simulink model "particle_fluid_surface_interaction_model"  (R2024b)
settings: Solver=ode4  StartTime=0.0  StopTime=params.tEnd  FixedStep=params.dt  RelTol=1e-3
undefined symbols (not defined in the file): params
libraries: slpidlib x1
settings Model: Creator=nihalseth34  LastModifiedBy=nihalseth34
settings DebuggingCC: AlgebraicLoopMsg=none  IgnoredZcDiagnostic=none

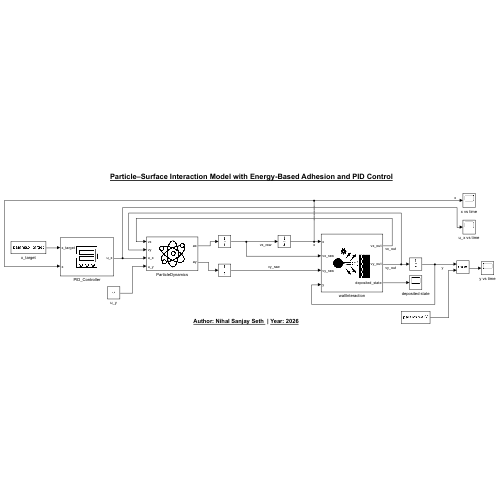
[thumbnail: Simulink's stored preview of the top-level diagram]
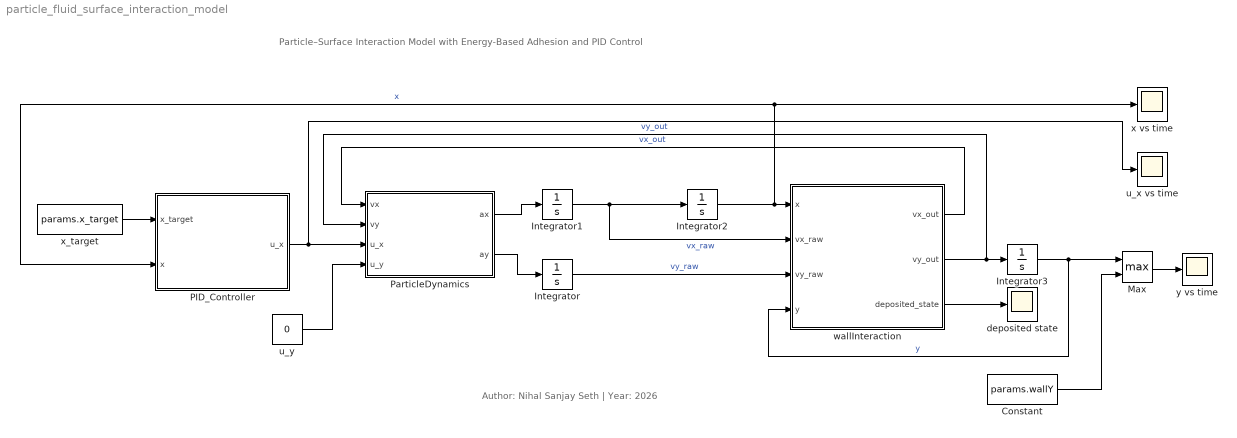
== system particle_fluid_surface_interaction_model ==
  note: Author: Nihal Sanjay Seth | Year: 2026
  note: Particle–Surface Interaction Model with Energy-Based Adhesion and PID Control
  Constant : Constant  Value=params.wallY
  Integrator : Integrator  ZeroCross=off
  Integrator1 : Integrator  InitialCondition=1
  Integrator2 : Integrator
  Integrator3 : Integrator  InitialCondition=1
  Max : MinMax  Function=max  Inputs=2
  PID_Controller : Subsystem
      mask Display: image('mask_images\PID_controller.png', [0,0,0,0,80,80]);
  ParticleDynamics : Subsystem
      mask Display: image('mask_images\ParticleDynamics.png', [0,0,0,0,80,80]);
  deposited state : Scope
  u_x vs time : Scope
  u_y : Constant  Value=0
  wallInteraction : Subsystem
      mask Display: image('mask_images\wallInteraction.png', [0,0,0,0,80,80]);
  x vs time : Scope
  x_target : Constant  Value=params.x_target
  y vs time : Scope
  wires:
  Integrator1/1 -> wallInteraction/2(vx_raw), Integrator2/1  "vx_raw"
  Integrator/1 -> wallInteraction/3(vy_raw)  "vy_raw"
  ParticleDynamics/1(ax) -> Integrator1/1
  ParticleDynamics/2(ay) -> Integrator/1
  Integrator2/1 -> x vs time/1, PID_Controller/2(x), wallInteraction/1(x)  "x"
  wallInteraction/1(vx_out) -> ParticleDynamics/1(vx)  "vx_out"
  wallInteraction/3(deposited_state) -> deposited state/1
  PID_Controller/1(u_x) -> u_x vs time/1, ParticleDynamics/3(u_x)
  x_target/1 -> PID_Controller/1(x_target)
  u_y/1 -> ParticleDynamics/4(u_y)
  wallInteraction/2(vy_out) -> Integrator3/1, ParticleDynamics/2(vy)  "vy_out"
  Integrator3/1 -> Max/1, wallInteraction/4(y)  "y"
  Max/1 -> y vs time/1
  Constant/1 -> Max/2

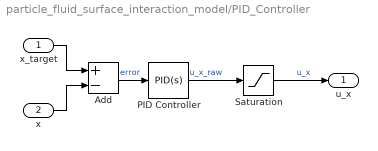
== system particle_fluid_surface_interaction_model/PID_Controller ==
  x_target : Inport
  x : Inport  Port=2
  Add : Sum  Inputs=+-
  PID Controller : slpidlib/PID Controller  Controller=PID  Form=Parallel  TimeDomain=Continuous-time  UseExternalTs=off  SampleTime=params.dt  IntegratorMethod=Forward Euler  FilterMethod=Forward Euler  ControllerParametersSource=internal  P=params.Kp  I=params.Ki  UseKiTs=off  D=params.Kd  UseExternalDerivativeSource=off  N=100  UseFilter=on  TunerSelectOption=Transfer Function Based (PID Tuner App)  InitialConditionSource=internal  InitialConditionForIntegrator=0  InitialConditionForFilter=0  DifferentiatorICPrevScaledInput=0  ExternalReset=none  TrackingMode=off  Kt=1  LimitOutput=off  SatLimitsSource=internal  UpperSaturationLimit=inf  LowerSaturationLimit=-inf  LinearizeAsGain=on  AntiWindupMode=none  Kb=1  LimitIntegrator=off  UpperIntegratorSaturationLimit=inf  LowerIntegratorSaturationLimit=-inf  POutMin=[]  POutMax=[]  IOutMin=[]  IOutMax=[]  DOutMin=[]  DOutMax=[]  NOutMin=[]  NOutMax=[]  SumOutMin=[]  SumOutMax=[]  SaturationOutMin=[]  SaturationOutMax=[]  PParamMin=[]  PParamMax=[]  IParamMin=[]  IParamMax=[]  DParamMin=[]  DParamMax=[]  NParamMin=[]  NParamMax=[]  KbParamMin=[]  KbParamMax=[]  KtParamMin=[]  KtParamMax=[]  KbOutMin=[]  KbOutMax=[]  KtOutMin=[]  KtOutMax=[]  IntegratorOutMin=[]  IntegratorOutMax=[]  FilterOutMin=[]  FilterOutMax=[]  SumI1OutMin=[]  SumI1OutMax=[]  SumI2OutMin=[]  SumI2OutMax=[]  SumI3OutMin=[]  SumI3OutMax=[]  SumI4OutMin=[]  SumI4OutMax=[]  SumDOutMin=[]  SumDOutMax=[]  DifferentiatorOutMin=[]  DifferentiatorOutMax=[]  FilterDiffOutCoefMin=[]  FilterDiffOutCoefMax=[]  ReciprocalOutMin=[]  ReciprocalOutMax=[]  SumDenOutMin=[]  SumDenOutMax=[]  SumNumOutMin=[]  SumNumOutMax=[]  DivideOutMin=[]  DivideOutMax=[]  UdiffTsProdOutMin=[]  UdiffTsProdOutMax=[]  NTsProdOutMin=[]  NTsProdOutMax=[]  UintegralTsProdOutMin=[]  UintegralTsProdOutMax=[]  UngainTsProdOutMin=[]  UngainTsProdOutMax=[]  ClampingZeroOutDataTypeStr=Inherit: Inherit via back propagation  ClampingZeroOutMin=[]  ClampingZeroOutMax=[]  FilterDenConstantOutDataTypeStr=Inherit: Inherit via back propagation  FilterDenConstantOutMin=[]  FilterDenConstantOutMax=[]  PCopyOutDataTypeStr=Inherit: Inherit via back propagation  PCopyOutMin=[]  PCopyOutMax=[]  NCopyOutDataTypeStr=Inherit: Inherit via back propagation  NCopyOutMin=[]  NCopyOutMax=[]  IntegratorContinuousStateAttributes=''  IntegratorStateMustResolveToSignalObject=off  IntegratorRTWStateStorageClass=Auto  FilterContinuousStateAttributes=''  FilterStateMustResolveToSignalObject=off  FilterRTWStateStorageClass=Auto  ParallelPVariant=InternalParameters  IdealPVariant=Disabled  IVariant=InternalParameters  DVariant=InternalParameters  IntegratorVariant=Continuous  SatVariant=Disabled  AWVariant=Passthrough  PCopyVariant=Disabled  TRVariant=Disabled  FdbkBlocksVariant=Forward  IdealPFdbkVariant=Disabled  SatFdbkVariant=Disabled  DerivativeFilterVariant=ContFilter  NVariant=InternalParameters  NCopyVariant=Disabled  FilterICVariant=InternalICsFilter  IntegratorICVariant=InternalICs  ExternalResetVariant=Disabled  TRSumVariant=Passthrough  SumFdbkVariant=Disabled  SumVariant=Sum_PID  TsampFilterVariant=InternalTs  TsampNgainVariant=Passthrough  TsampIntegralVariant=Disabled_SignalSpec  ExternalSaturationOutDataTypeStr=Inherit: Same as second input  DerivativeSourceVariant=ErrorSignal  PreIntVariant=InternalPreInt
  Saturation : Saturate  UpperLimit=params.u_max  LowerLimit=-params.u_max
  u_x : Outport
  wires:
  x_target/1 -> Add/1
  x/1 -> Add/2
  Add/1 -> PID Controller/1  "error"
  PID Controller/1 -> Saturation/1  "u_x_raw"
  Saturation/1 -> u_x/1  "u_x"

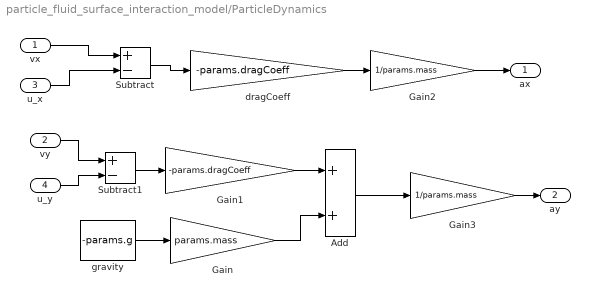
== system particle_fluid_surface_interaction_model/ParticleDynamics ==
  vx : Inport
  vy : Inport  Port=2
  u_x : Inport  Port=3
  u_y : Inport  Port=4
  Add : Sum
  Gain : Gain  Gain=params.mass
  Gain1 : Gain  Gain=-params.dragCoeff
  Gain2 : Gain  Gain=1/params.mass
  Gain3 : Gain  Gain=1/params.mass
  Subtract : Sum  Inputs=+-
  Subtract1 : Sum  Inputs=+-
  dragCoeff : Gain  Gain=-params.dragCoeff
  gravity : Constant  Value=-params.g
  ax : Outport
  ay : Outport  Port=2
  wires:
  vy/1 -> Subtract1/1
  u_x/1 -> Subtract/2
  u_y/1 -> Subtract1/2
  vx/1 -> Subtract/1
  Subtract/1 -> dragCoeff/1
  dragCoeff/1 -> Gain2/1
  Subtract1/1 -> Gain1/1
  Gain1/1 -> Add/1
  Gain2/1 -> ax/1
  gravity/1 -> Gain/1
  Gain3/1 -> ay/1
  Gain/1 -> Add/2
  Add/1 -> Gain3/1

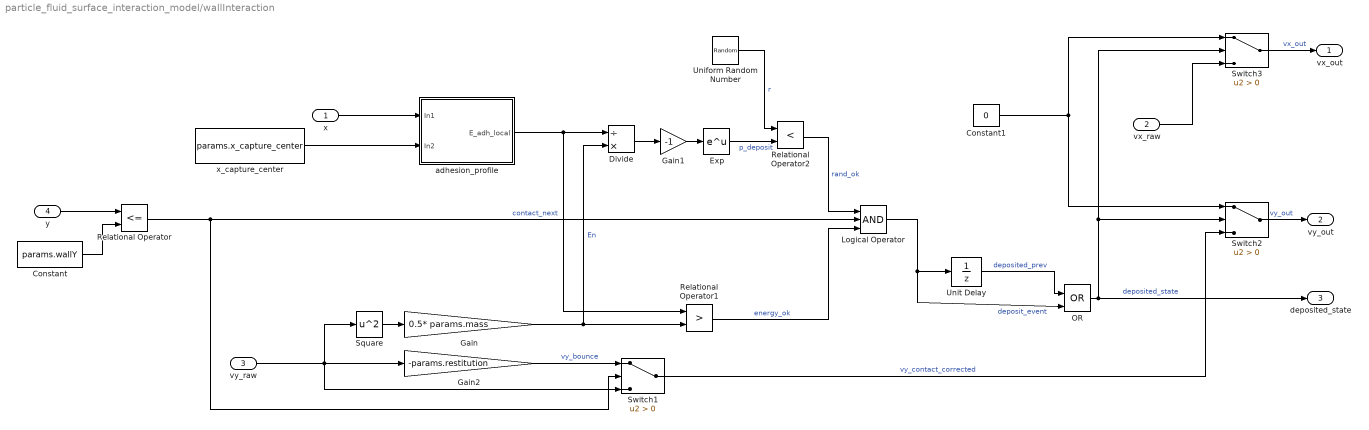
== system particle_fluid_surface_interaction_model/wallInteraction ==
  x : Inport
  vx_raw : Inport  Port=2
  vy_raw : Inport  Port=3
  y : Inport  Port=4
  Constant : Constant  Value=params.wallY
  Constant1 : Constant  Value=0
  Divide : Product  Inputs=/*
  Exp : Math
  Gain : Gain  Gain=0.5* params.mass
  Gain1 : Gain  Gain=-1
  Gain2 : Gain  Gain=-params.restitution
  Logical Operator : Logic  Inputs=3  AllPortsSameDT=off  OutDataTypeStr=boolean
  OR : Logic  Operator=OR  IconShape=distinctive  AllPortsSameDT=off  OutDataTypeStr=boolean
  Relational Operator : RelationalOperator  Operator=<=  OutDataTypeStr=boolean  RndMeth=Simplest  InputSameDT=off
  Relational Operator1 : RelationalOperator  Operator=>  OutDataTypeStr=boolean  RndMeth=Simplest  InputSameDT=off
  Relational Operator2 : RelationalOperator  Operator=<  OutDataTypeStr=boolean  RndMeth=Simplest  InputSameDT=off
  Square : Math  Operator=square
  Switch1 : Switch  Criteria=u2 > Threshold  SaturateOnIntegerOverflow=off  InputSameDT=off
  Switch2 : Switch  Criteria=u2 > Threshold  SaturateOnIntegerOverflow=off  InputSameDT=off
  Switch3 : Switch  Criteria=u2 > Threshold  SaturateOnIntegerOverflow=off  InputSameDT=off
  Uniform Random Number : UniformRandomNumber  Minimum=0  SampleTime=0.01
  Unit Delay : UnitDelay  SampleTime=-1  HasFrameUpgradeWarning=on
  adhesion_profile : Subsystem
  x_capture_center : Constant  Value=params.x_capture_center
  vx_out : Outport
  vy_out : Outport  Port=2
  deposited_state : Outport  Port=3
  wires:
  vy_raw/1 -> Switch1/3, Gain2/1, Square/1
  Divide/1 -> Gain1/1
  OR/1 -> Switch3/2, Switch2/2, deposited_state/1  "deposited_state"
  Relational Operator1/1 -> Logical Operator/3  "energy_ok"
  Constant/1 -> Relational Operator/2
  Gain1/1 -> Exp/1
  Gain/1 -> Divide/2, Relational Operator1/2  "En"
  Switch2/1 -> vy_out/1  "vy_out"
  Relational Operator2/1 -> Logical Operator/1  "rand_ok"
  Gain2/1 -> Switch1/1  "vy_bounce"
  Square/1 -> Gain/1
  Switch1/1 -> Switch2/3  "vy_contact_corrected"
  Exp/1 -> Relational Operator2/2  "p_deposit"
  y/1 -> Relational Operator/1
  Logical Operator/1 -> OR/2, Unit Delay/1  "deposit_event"
  Constant1/1 -> Switch3/1, Switch2/1
  vx_raw/1 -> Switch3/3
  Uniform Random Number/1 -> Relational Operator2/1  "r"
  Switch3/1 -> vx_out/1  "vx_out"
  Unit Delay/1 -> OR/1  "deposited_prev"
  Relational Operator/1 -> Logical Operator/2, Switch1/2  "contact_next"
  adhesion_profile/1(E_adh_local) -> Divide/1, Relational Operator1/1
  x/1 -> adhesion_profile/1(In1)
  x_capture_center/1 -> adhesion_profile/2(In2)

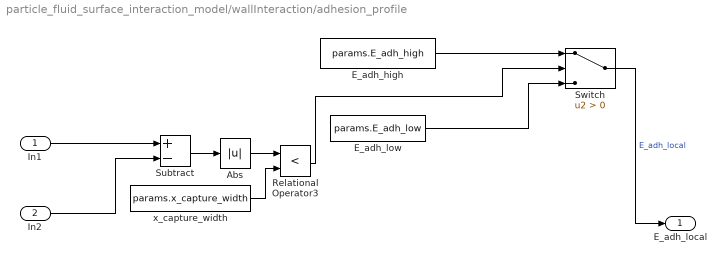
== system particle_fluid_surface_interaction_model/wallInteraction/adhesion_profile ==
  In1 : Inport
  In2 : Inport  Port=2
  Abs : Abs  SaturateOnIntegerOverflow=off
  E_adh_high : Constant  Value=params.E_adh_high
  E_adh_low : Constant  Value=params.E_adh_low
  Relational Operator3 : RelationalOperator  Operator=<  OutDataTypeStr=boolean  RndMeth=Simplest  InputSameDT=off
  Subtract : Sum  Inputs=+-
  Switch : Switch  Criteria=u2 > Threshold  SaturateOnIntegerOverflow=off  InputSameDT=off
  x_capture_width : Constant  Value=params.x_capture_width
  E_adh_local : Outport
  wires:
  x_capture_width/1 -> Relational Operator3/2
  Subtract/1 -> Abs/1
  E_adh_high/1 -> Switch/1
  Abs/1 -> Relational Operator3/1
  In1/1 -> Subtract/1
  E_adh_low/1 -> Switch/3
  In2/1 -> Subtract/2
  Relational Operator3/1 -> Switch/2
  Switch/1 -> E_adh_local/1  "E_adh_local"
